simulink model "UnitDelay2"  (R2020a)
settings: Solver=VariableStepAuto  StartTime=0.0  StopTime=10.0  RelTol=1e-3
settings Model: Creator=bzhan  LastModifiedBy=bzhan

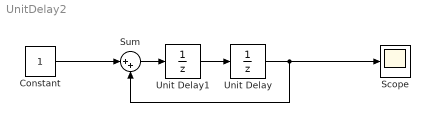
== system UnitDelay2 ==
  Constant : Constant
  Scope : Scope
  Sum : Sum  Inputs=|++
  Unit Delay : UnitDelay  SampleTime=-1  HasFrameUpgradeWarning=on
  Unit Delay1 : UnitDelay  SampleTime=-1  HasFrameUpgradeWarning=on
  wires:
  Constant/1 -> Sum/1
  Unit Delay/1 -> Scope/1, Sum/2
  Sum/1 -> Unit Delay1/1
  Unit Delay1/1 -> Unit Delay/1
